simulink model "SVM_Low_Level"  (R2021a)
settings: Solver=ode23s  StartTime=0.0  StopTime=.02*20  MaxStep=1e-4  RelTol=1e-3
model workspace (MAT data in the model file):
  time_sample = 0.0001
undefined symbols (not defined in the file): Down, Up
libraries: spsIGBTDiodeLib x12, eePwmGenerator x6, spsThreePhaseVIMeasurementLib x3, dsparch4 x2, spsDCVoltageSourceLib x2, spsRMSLib x2, simulink x2, spsVoltageMeasurementLib x2, spsAsynchronousMachineSIUnitsLib x1, spsGroundLib x1, spsThreePhaseSeriesRLCBranchLib x1, spspowerguiLib x1
settings Model: Creator=Ahmed Mohamed  LastModifiedBy=Ahmed Mohamed
settings DataIOCC: ReturnWorkspaceOutputs=off

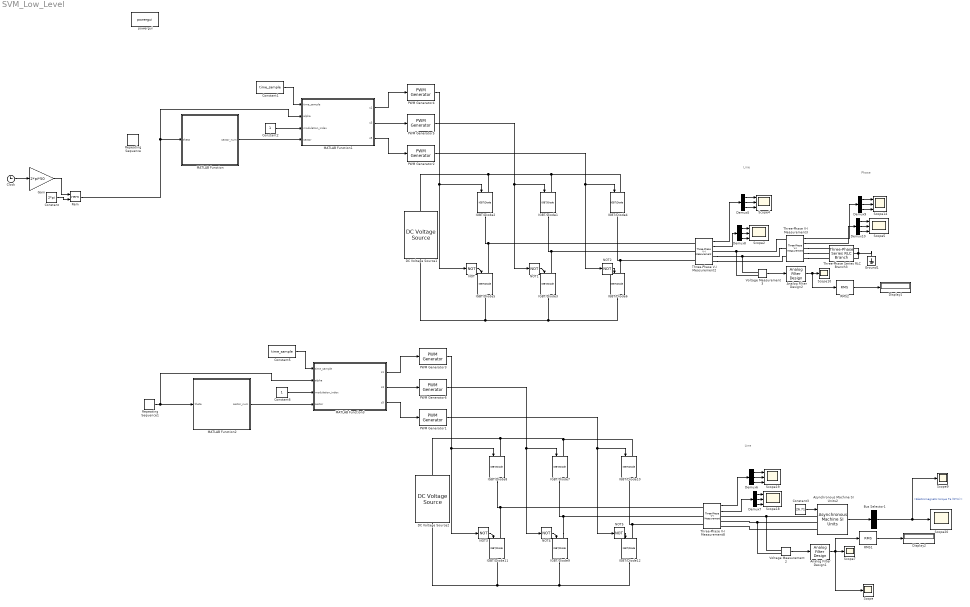
== system SVM_Low_Level ==
  note: Phase
  note: Line
  note: Line
  Analog Filter Design1 : dsparch4/Analog Filter Design  method=Butterworth  filttype=Lowpass  N=8  Wlo=2*pi*1000  Whi=80  Rp=2  Rs=40
  Analog Filter Design2 : dsparch4/Analog Filter Design  method=Butterworth  filttype=Lowpass  N=8  Wlo=2*pi*1000  Whi=80  Rp=2  Rs=40
  Asynchronous Machine SI Units2 : spsAsynchronousMachineSIUnitsLib/Asynchronous Machine SI Units  RotorType=Squirrel-cage  PresetModel="15:  5.4 HP (4KW)   400 V  50Hz 1430 RPM"  MechanicalLoad=Torque Tm  ShowDetailedParameters=on  ReferenceFrame=Rotor  Units=SI  MeasurementBus=off  NominalParameters=[4000 400 50]  VoltageRatio=1  Stator=[1.405 0.005839]  Rotor=[1.395 0.005839]  Cage1=[0.4155 0.002066]  Cage2=[0.4168 0.0003495]  Lm=0.1722  Mechanical=[0.0131 0.002985 2]  PolePairs=2  InitialConditions=[1 0 0 0 0 0 0 0]  SimulateSaturation=off  Saturation=[14.03593122, 27.81365428, 53.79336849, 72.68890987, 97.98006896, 148.6815601, 215.7428561, 302.9841135, 428.7778367 ; 230, 322, 414, 460, 506, 552, 598, 644, 690]  LoadFlowParameters=1492000  TsPowergui=0  TsBlock=-1  IterativeModel=Trapezoidal non iterative  IterativeDiscreteModel=Trapezoidal non iterative  Pmec=1.492e+006
  Bus Selector1 : BusSelector  OutputSignals=Mechanical.Electromagnetic torque Te (N*m)
  Clock : Clock
  Constant : Constant  Value=2*pi
  Constant1 : Constant  Value=time_sample
  Constant2 : Constant
  Constant3 : Constant  Value=26.71
  Constant5 : Constant  Value=time_sample
  Constant6 : Constant
  DC Voltage Source1 : spsDCVoltageSourceLib/DC Voltage Source  Amplitude=570  Measurements=None
  DC Voltage Source2 : spsDCVoltageSourceLib/DC Voltage Source  Amplitude=570  Measurements=None
  Demux{5..10} (6 alike) : Demux  Outputs=3
  Display1 : Display
  Display2 : Display
  Gain : Gain  Gain=2*pi*50
  Ground1 : spsGroundLib/Ground  LConnTagsString=a
  IGBT/Diode{1..12} (12 alike) : spsIGBTDiodeLib/IGBT//Diode  Ron=1e-3  Rs=1e5  Cs=inf  Measurements=off
  MATLAB Function : MATLAB Function  TreatAsAtomicUnit=on
  MATLAB Function1 : MATLAB Function  TreatAsAtomicUnit=on
  MATLAB Function2 : MATLAB Function  TreatAsAtomicUnit=on
  MATLAB Function3 : MATLAB Function  TreatAsAtomicUnit=on
  NOT{,1..5} (6 alike) : Logic  Operator=NOT  IconShape=distinctive  AllPortsSameDT=off  OutDataTypeStr=boolean
  PWM Generator{1..6} (6 alike) : eePwmGenerator/PWM Generator  CarrCount=Up-Down  Tper=time_sample*.5  Ts=1e-6
  RMS1 : spsRMSLib/RMS  TrueRMS=off  Freq=50  RMSInit=0  Ts=0
  RMS2 : spsRMSLib/RMS  TrueRMS=off  Freq=50  RMSInit=0  Ts=0
  Rem : Math  Operator=rem  SaturateOnIntegerOverflow=on
  Repeating Sequence : simulink/Sources/Repeating Sequence  rep_seq_t=[0 .02]  rep_seq_y=[0 2*pi]
  Repeating Sequence1 : simulink/Sources/Repeating Sequence  rep_seq_t=[0 .02]  rep_seq_y=[0 2*pi]
  Scope{,7,9..10,20} (5 alike) : Scope
  Scope{2,4..5,14,18..19} (6 alike) : Scope  NumInputPorts=3
  Three-Phase Series RLC Branch3 : spsThreePhaseSeriesRLCBranchLib/Three-Phase Series RLC Branch  LConnTagsString=A|B|C  RConnTagsString=A|B|C  BranchType=RL  Resistance=7.5*sqrt(2)  Inductance=7.5*sqrt(2)/314  Capacitance=1e-6  Measurements=None
  Three-Phase V-I Measurement2 : spsThreePhaseVIMeasurementLib/Three-Phase V-I Measurement  VoltageMeasurement=phase-to-phase  SetLabelV=off  LabelV=Vabc  Vpu=off  VpuLL=off  CurrentMeasurement=yes  SetLabelI=off  LabelI=Iabc  Ipu=off  Pbase=100e6  Vbase=500e3  OutputType=Complex  PhasorSimulation=off  PSBequivalent=0
  Three-Phase V-I Measurement3 : spsThreePhaseVIMeasurementLib/Three-Phase V-I Measurement  VoltageMeasurement=phase-to-ground  SetLabelV=off  LabelV=Vabc  Vpu=off  VpuLL=off  CurrentMeasurement=yes  SetLabelI=off  LabelI=Iabc  Ipu=off  Pbase=100e6  Vbase=500e3  OutputType=Complex  PhasorSimulation=off  PSBequivalent=0
  Three-Phase V-I Measurement8 : spsThreePhaseVIMeasurementLib/Three-Phase V-I Measurement  VoltageMeasurement=phase-to-phase  SetLabelV=off  LabelV=Vabc  Vpu=off  VpuLL=off  CurrentMeasurement=yes  SetLabelI=off  LabelI=Iabc  Ipu=off  Pbase=100e6  Vbase=500e3  OutputType=Complex  PhasorSimulation=off  PSBequivalent=0
  Voltage Measurement2 : spsVoltageMeasurementLib/Voltage Measurement  PhasorSimulation=off  OutputType=Complex  PSBequivalent=0
  Voltage Measurement3 : spsVoltageMeasurementLib/Voltage Measurement  PhasorSimulation=off  OutputType=Complex  PSBequivalent=0
  powergui : spspowerguiLib/powergui  Priority=1  SimulationMode=Discrete  SampleTime=1e-6  frequency=60  Iterations=50  frequencyindice=0  Pbase=100e6  ErrMax=1e-4  UnitsV=kV  UnitsW=MW  buscounter=0  FunctionMessages=off  echomessages=off  EnableUseOfTLC=off  CurrentSourceSwitches=off  DisableSnubberDevices=off  DisableRonSwitches=off  DisableVfSwitches=off  DisplayEquations=off  AutomaticDiscreteSolvers=off  SolverType=Tustin/Backward Euler (TBE)  Interpol=off  ExternalGateDelay=off  methode=off  Ts=100  x0status=blocks  SPID=on  SwTol=0  HookPort=off  NonlinearTolerance=1e-4  nMaxIteration=100  ContinueOnMaxIteration=off  RestoreLinks=warning  ResistiveCurrentMeasurement=off  Frange=[0:2:500]  Ylog=off  Xlog=on  ShowGrid=off  save=off  variable=ZData  structure=0  ZoomFFT=off  StartTime=0.0  cycles=1  DisplayStyle=1  fundamental=60  FreqAxis=off  MaxFrequency=1000  frequencyindicesteady=1  RmsSteady=1  display=off
  wires:
  Constant1/1 -> MATLAB Function1/1(time_sample)
  MATLAB Function/1(sector_num) -> MATLAB Function1/4(sector)
  Constant2/1 -> MATLAB Function1/3(modulation_index)
  NOT1/1 -> IGBT/Diode3/1
  PWM Generator5/1 -> NOT1/1, IGBT/Diode1/1
  NOT/1 -> IGBT/Diode5/1
  PWM Generator4/1 -> NOT/1, IGBT/Diode2/1
  PWM Generator2/1 -> NOT2/1, IGBT/Diode4/1
  NOT2/1 -> IGBT/Diode6/1
  MATLAB Function1/1(s1) -> PWM Generator4/1
  MATLAB Function1/2(s3) -> PWM Generator5/1
  MATLAB Function1/3(s5) -> PWM Generator2/1
  Clock/1 -> Gain/1
  Gain/1 -> Rem/1
  Constant/1 -> Rem/2
  RMS2/1 -> Display1/1
  Voltage Measurement3/1 -> Analog Filter Design2/1
  Three-Phase V-I Measurement3/2 -> Demux10/1
  Demux8/2 -> Scope2/2
  Demux10/2 -> Scope5/2
  Three-Phase V-I Measurement3/1 -> Demux9/1
  Analog Filter Design2/1 -> Scope10/1, RMS2/1
  Demux5/1 -> Scope4/1
  Demux8/3 -> Scope2/3
  Demux9/1 -> Scope14/1
  Demux5/2 -> Scope4/2
  Demux10/3 -> Scope5/3
  Demux9/3 -> Scope14/3
  Three-Phase V-I Measurement2/1 -> Demux5/1
  Three-Phase V-I Measurement2/2 -> Demux8/1
  Demux8/1 -> Scope2/1
  Demux9/2 -> Scope14/2
  Demux5/3 -> Scope4/3
  Demux10/1 -> Scope5/1
  Asynchronous Machine SI Units2/1 -> Bus Selector1/1
  RMS1/1 -> Display2/1
  Analog Filter Design1/1 -> RMS1/1, Scope/1, Scope7/1
  Constant3/1 -> Asynchronous Machine SI Units2/1
  Demux7/1 -> Scope18/1
  Demux6/1 -> Scope19/1
  Demux7/2 -> Scope18/2
  Voltage Measurement2/1 -> Analog Filter Design1/1
  Demux6/3 -> Scope19/3
  Three-Phase V-I Measurement8/2 -> Demux7/1
  Demux6/2 -> Scope19/2
  Demux7/3 -> Scope18/3
  Bus Selector1/1 -> Scope9/1, Scope20/1  "<Electromagnetic torque Te (N*m)>"
  Three-Phase V-I Measurement8/1 -> Demux6/1
  Repeating Sequence1/1 -> MATLAB Function3/2(alpha), MATLAB Function2/1(theta)
  MATLAB Function3/3(s5) -> PWM Generator1/1
  MATLAB Function3/2(s3) -> PWM Generator6/1
  MATLAB Function3/1(s1) -> PWM Generator3/1
  NOT5/1 -> IGBT/Diode12/1
  PWM Generator1/1 -> IGBT/Diode10/1, NOT5/1
  PWM Generator3/1 -> IGBT/Diode8/1, NOT3/1
  NOT3/1 -> IGBT/Diode11/1
  PWM Generator6/1 -> IGBT/Diode7/1, NOT4/1
  NOT4/1 -> IGBT/Diode9/1
  Constant6/1 -> MATLAB Function3/3(modulation_index)
  MATLAB Function2/1(sector_num) -> MATLAB Function3/4(sector)
  Constant5/1 -> MATLAB Function3/1(time_sample)
  Rem/1 -> MATLAB Function1/2(alpha), MATLAB Function/1(theta)
  connections:
  IGBT/Diode2/RConn1 -- Three-Phase V-I Measurement2/LConn1 -- IGBT/Diode5/LConn1
  IGBT/Diode1/LConn1 -- DC Voltage Source1/RConn1 -- IGBT/Diode2/LConn1 -- IGBT/Diode4/LConn1
  IGBT/Diode1/RConn1 -- Three-Phase V-I Measurement2/LConn2 -- IGBT/Diode3/LConn1
  IGBT/Diode6/LConn1 -- Three-Phase V-I Measurement2/LConn3 -- IGBT/Diode4/RConn1
  IGBT/Diode3/RConn1 -- IGBT/Diode6/RConn1 -- DC Voltage Source1/LConn1 -- IGBT/Diode5/RConn1
  Three-Phase V-I Measurement2/RConn1 -- Three-Phase V-I Measurement3/LConn1 -- Voltage Measurement3/LConn2
  Ground1/LConn1 -- Three-Phase Series RLC Branch3/RConn2 -- Three-Phase Series RLC Branch3/RConn3 -- Three-Phase Series RLC Branch3/RConn1
  Three-Phase V-I Measurement3/LConn2 -- Three-Phase V-I Measurement2/RConn2 -- Voltage Measurement3/LConn1
  Three-Phase V-I Measurement2/RConn3 -- Three-Phase V-I Measurement3/LConn3
  Three-Phase V-I Measurement3/RConn1 -- Three-Phase Series RLC Branch3/LConn1
  Three-Phase V-I Measurement3/RConn3 -- Three-Phase Series RLC Branch3/LConn3
  Three-Phase V-I Measurement3/RConn2 -- Three-Phase Series RLC Branch3/LConn2
  Three-Phase V-I Measurement8/RConn2 -- Asynchronous Machine SI Units2/LConn2 -- Voltage Measurement2/LConn2
  Three-Phase V-I Measurement8/RConn1 -- Asynchronous Machine SI Units2/LConn1 -- Voltage Measurement2/LConn1
  Asynchronous Machine SI Units2/LConn3 -- Three-Phase V-I Measurement8/RConn3
  IGBT/Diode8/RConn1 -- Three-Phase V-I Measurement8/LConn1 -- IGBT/Diode11/LConn1
  DC Voltage Source2/RConn1 -- IGBT/Diode8/LConn1 -- IGBT/Diode7/LConn1 -- IGBT/Diode10/LConn1
  IGBT/Diode9/LConn1 -- Three-Phase V-I Measurement8/LConn2 -- IGBT/Diode7/RConn1
  IGBT/Diode10/RConn1 -- Three-Phase V-I Measurement8/LConn3 -- IGBT/Diode12/LConn1
  IGBT/Diode12/RConn1 -- IGBT/Diode9/RConn1 -- IGBT/Diode11/RConn1 -- DC Voltage Source2/LConn1

== matlab function SVM_Low_Level/MATLAB Function1 ==
  data: time_sample input; s1 output; alpha input; modulation_index input; s3 output; s5 output; sector input
function [s1, s3, s5] = calcDutyCycle(time_sample, alpha, modulation_index, sector)
theta_prime = alpha-(pi/3)*(sector-1);
ta = modulation_index * time_sample*sin((pi/3)-theta_prime);
tb = modulation_index * time_sample*sin(theta_prime);
to = time_sample - ta - tb;

X_duty_cycle = (.5*to+ta+tb)/time_sample;
Y2_duty_cycle = (.5*to+ta)/time_sample;
Y1_duty_cycle = (.5*to+tb)/time_sample;
Z_duty_cycle = (.5*to)/time_sample;
switch(sector)
    case(1)
       s1 =  X_duty_cycle;
       s3 =  Y1_duty_cycle;
       s5 = Z_duty_cycle;
    case(2)
       s1 =  Y2_duty_cycle;
       s3 =  X_duty_cycle;
       s5 =  Z_duty_cycle;
    case(3)
       s1 =  Z_duty_cycle;
       s3 =  X_duty_cycle;
       s5 =  Y1_duty_cycle;
    case(4)
       s1 =  Z_duty_cycle;
       s3 =  Y2_duty_cycle;
       s5 =  X_duty_cycle;
    case(5)
       s1 =  Y1_duty_cycle;
       s3 =  Z_duty_cycle;
       s5 = X_duty_cycle;
    case(6)
       s1 =  X_duty_cycle;
       s3 =  Z_duty_cycle;
       s5 =  Y2_duty_cycle;
    otherwise
        s1 = 0;
        s3 = 0;
        s5 = 0;
end

== matlab function SVM_Low_Level/MATLAB Function ==
  data: theta input; sector_num output
function sector_num = get_sector_number(theta)
if (theta>=0 && theta <(pi/3)) 
    sector_num = 1;
elseif (theta >=(1*pi/3) && theta<(2*pi/3)) 
    sector_num = 2;
elseif (theta >=(2*pi/3) && theta<(3*pi/3)) 
    sector_num = 3;
elseif (theta >=(3*pi/3) && theta<(4*pi/3)) 
    sector_num = 4;
elseif (theta >=(4*pi/3) && theta<(5*pi/3)) 
    sector_num = 5;
else
    sector_num = 6;
end

== matlab function SVM_Low_Level/MATLAB Function2 ==
  data: theta input; sector_num output
function sector_num = get_sector_number(theta)
if (theta>=0 && theta <(pi/3)) 
    sector_num = 1;
elseif (theta >=(1*pi/3) && theta<(2*pi/3)) 
    sector_num = 2;
elseif (theta >=(2*pi/3) && theta<(3*pi/3)) 
    sector_num = 3;
elseif (theta >=(3*pi/3) && theta<(4*pi/3)) 
    sector_num = 4;
elseif (theta >=(4*pi/3) && theta<(5*pi/3)) 
    sector_num = 5;
else
    sector_num = 6;
end

== matlab function SVM_Low_Level/MATLAB Function3 ==
  data: time_sample input; s1 output; alpha input; modulation_index input; s3 output; s5 output; sector input
function [s1, s3, s5] = fcn(time_sample, alpha, modulation_index, sector)


theta_prime = alpha-(pi/3)*(sector-1);
ta = modulation_index * time_sample*sin((pi/3)-theta_prime);
tb = modulation_index * time_sample*sin(theta_prime);

%ta = sqrt(3)*time_sample*((V_d/sqrt(3))/V_d)*sin((pi/3)-(alpha-(pi/3)*(sector-1));

% tb = time_sample * modulation_index * sin((alpha-(sector-1)*pi/3));
to = time_sample - ta - tb;

X_duty_cycle = (.5*to+ta+tb)/time_sample;
Y2_duty_cycle = (.5*to+ta)/time_sample;
Y1_duty_cycle = (.5*to+tb)/time_sample;
Z_duty_cycle = (.5*to)/time_sample;
switch(sector)
    case(1)
       s1 =  X_duty_cycle;
       s3 =  Y1_duty_cycle;
       s5 = Z_duty_cycle;
    case(2)
       s1 =  Y2_duty_cycle;
       s3 =  X_duty_cycle;
       s5 =  Z_duty_cycle;
    case(3)
       s1 =  Z_duty_cycle;
       s3 =  X_duty_cycle;
       s5 =  Y1_duty_cycle;
    case(4)
       s1 =  Z_duty_cycle;
       s3 =  Y2_duty_cycle;
       s5 =  X_duty_cycle;
    case(5)
       s1 =  Y1_duty_cycle;
       s3 =  Z_duty_cycle;
       s5 = X_duty_cycle;
    case(6)
       s1 =  X_duty_cycle;
       s3 =  Z_duty_cycle;
       s5 =  Y2_duty_cycle;
    otherwise
        s1 = 0;
        s3 = 0;
        s5 = 0;
end
